simulink model "adaptive_sliding_mode_controller_computed_torque"  (R2020a)
settings: Solver=ode1  StartTime=0.0  StopTime=50  FixedStep=0.01  RelTol=1e-3
model workspace (MAT data in the model file):
  kd = 0
  kp = 0
libraries: simulink x19, sharedutil x14, aerolibutil x4
(part 1 of 2)
settings Model: Creator=Sebas  LastModifiedBy=Sebas
settings SolverCC: ZeroCrossAlgorithm=Adaptive
settings DebuggingCC: MaskedZcDiagnostic=none  IgnoredZcDiagnostic=none

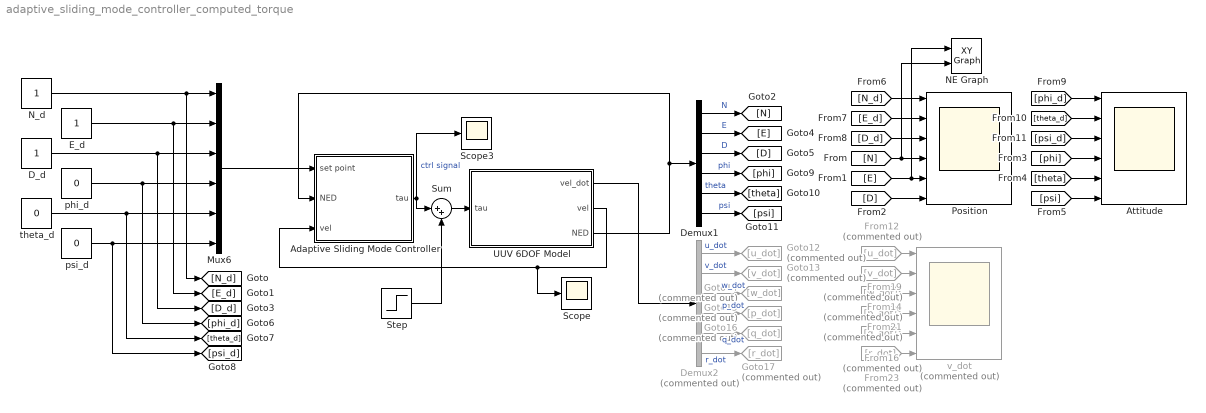
== system adaptive_sliding_mode_controller_computed_torque ==
  Adaptive Sliding Mode Controller : Subsystem
  Attitude : Scope  NumInputPorts=6
  D_d : Constant
  Demux1 : Demux  Outputs=6
  Demux2 : Demux  Commented=on  Outputs=6
  E_d : Constant
  From12 : From  Commented=on  GotoTag=u_dot
  From14 : From  Commented=on  GotoTag=w_dot
  From16 : From  Commented=on  GotoTag=q_dot
  From19 : From  Commented=on  GotoTag=v_dot
  From21 : From  Commented=on  GotoTag=p_dot
  From23 : From  Commented=on  GotoTag=r_dot
  Goto12 : Goto  Commented=on  GotoTag=u_dot
  Goto13 : Goto  Commented=on  GotoTag=v_dot
  Goto14 : Goto  Commented=on  GotoTag=w_dot
  Goto15 : Goto  Commented=on  GotoTag=p_dot
  Goto16 : Goto  Commented=on  GotoTag=q_dot
  Goto17 : Goto  Commented=on  GotoTag=r_dot
  Mux6 : Mux  Inputs=6
  NE Graph : simulink/Sinks/XY Graph  xmin=-1  xmax=5  ymin=-1  ymax=2  st=-1
  N_d : Constant
  Position : Scope  NumInputPorts=6
  Scope : Scope
  Scope3 : Scope
  Step : Step  Time=20  After=[30;30;30;5;5;5]  SampleTime=0
  Sum : Sum  Inputs=|++
  UUV 6DOF Model : Subsystem
  phi_d : Constant  Value=0
  psi_d : Constant  Value=0
  theta_d : Constant  Value=0
  v_dot : Scope  Commented=on  NumInputPorts=6
  wires:
  UUV 6DOF Model/3(NED) -> Adaptive Sliding Mode Controller/2(NED), Demux1/1
  Adaptive Sliding Mode Controller/1(tau) -> Sum/1, Scope3/1  "ctrl signal"
  [N_d] -> Position/1
  [E_d] -> Position/2
  [D_d] -> Position/3
  [N] -> Position/4, NE Graph/2
  [D] -> Position/6
  [E] -> Position/5, NE Graph/1
  Demux1/1 -> [N]  "N"
  Demux1/2 -> [E]  "E"
  Demux1/3 -> [D]  "D"
  [phi_d] -> Attitude/1
  [phi] -> Attitude/4
  [psi_d] -> Attitude/3
  [theta] -> Attitude/5
  [psi] -> Attitude/6
  [theta_d] -> Attitude/2
  Demux1/4 -> [phi]  "phi"
  Demux1/5 -> [theta]  "theta"
  Demux1/6 -> [psi]  "psi"
  UUV 6DOF Model/2(vel) -> Adaptive Sliding Mode Controller/3(vel), Scope/1
  UUV 6DOF Model/1(vel_dot) -> Demux2/1
  From12/1 -> v_dot/1
  From19/1 -> v_dot/2
  From14/1 -> v_dot/3
  From21/1 -> v_dot/4
  From16/1 -> v_dot/5
  From23/1 -> v_dot/6
  Demux2/1 -> Goto12/1  "u_dot"
  Demux2/5 -> Goto16/1  "q_dot"
  Demux2/3 -> Goto14/1  "w_dot"
  Demux2/6 -> Goto17/1  "r_dot"
  Demux2/4 -> Goto15/1  "p_dot"
  Demux2/2 -> Goto13/1  "v_dot"
  D_d/1 -> Mux6/3, [D_d]
  theta_d/1 -> [theta_d], Mux6/5
  Mux6/1 -> Adaptive Sliding Mode Controller/1(set point)
  phi_d/1 -> Mux6/4, [phi_d]
  E_d/1 -> [E_d], Mux6/2
  N_d/1 -> [N_d], Mux6/1
  psi_d/1 -> [psi_d], Mux6/6
  Sum/1 -> UUV 6DOF Model/1(tau)
  Step/1 -> Sum/2

== system adaptive_sliding_mode_controller_computed_torque/Adaptive Sliding Mode Controller ==
  set point : Inport
  NED : Inport  Port=2
  vel : Inport  Port=3
  ASMCs : Subsystem  Commented=on  mask(6 DOF Sliding Mode Controller){surge_k=10, sway_k=10, heave_k=2, roll_k=13, pitch_k=1, yaw_k=25, lambda=1, Kmin=0.001, k_alpha=0.002, miu=0.01}
      mask prompts: surge_k "Surge"; sway_k "Sway"; heave_k "Heave"; roll_k "Roll"; pitch_k "Pitch"; yaw_k "Yaw"
      mask help: Implementation of 6 Sliding Mode Controllers for each degree of freedom
      mask DialogControl ParameterGroupVar Prompt: K2 Gains
      mask DialogControl Container3 Prompt: Adaptation Law for K1
  ASMCs1 : Subsystem  Commented=on  mask(6 DOF Sliding Mode Controller){surge_k=3, sway_k=3, heave_k=1, roll_k=5, pitch_k=1, yaw_k=20, lambda=1, Kmin=0.005, k_alpha=0.0019, miu=0.01}
      mask prompts: surge_k "Surge"; sway_k "Sway"; heave_k "Heave"; roll_k "Roll"; pitch_k "Pitch"; yaw_k "Yaw"
      mask help: Implementation of 6 Sliding Mode Controllers for each degree of freedom
      mask DialogControl ParameterGroupVar Prompt: K2 Gains
      mask DialogControl Container3 Prompt: Adaptation Law for K1
  ASMCs2 : Subsystem  mask(6 DOF Sliding Mode Controller){surge_k=1, sway_k=1, heave_k=1, roll_k=5, pitch_k=1, yaw_k=20, lambda=1, Kmin=0.0001, k_alpha=0.1, miu=0.01}
      mask prompts: surge_k "Surge"; sway_k "Sway"; heave_k "Heave"; roll_k "Roll"; pitch_k "Pitch"; yaw_k "Yaw"
      mask help: Implementation of 6 Sliding Mode Controllers for each degree of freedom
      mask DialogControl ParameterGroupVar Prompt: K2 Gains
      mask DialogControl Container3 Prompt: Adaptation Law for K1
  NED to body : Subsystem
  Signal Specification : SignalSpecification  Dimensions=6
  Thrust allocation : Subsystem
  tau : Outport
  wires:
  NED to body/1(Out1) -> ASMCs2/1("position_d ")
  NED/1 -> NED to body/2(NED)
  Signal Specification/1 -> tau/1  "ideal"
  NED to body/2(Out2) -> ASMCs2/2(position)
  Thrust allocation/1(tau) -> Signal Specification/1
  ASMCs2/1(i_tau) -> Thrust allocation/1(ideal_tau)  "ideal_tau"
  vel/1 -> ASMCs2/3(vel)
  set point/1 -> NED to body/1(set point)

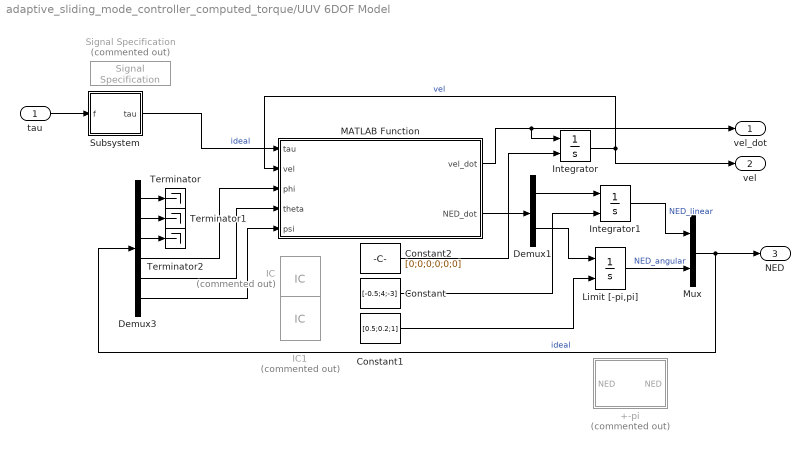
== system adaptive_sliding_mode_controller_computed_torque/UUV 6DOF Model ==
  tau : Inport
  +-pi : MATLAB Function  Commented=on  TreatAsAtomicUnit=on
  Constant : Constant  Value=[-0.5;4;-3]
  Constant1 : Constant  Value=[0.5;0.2;1]
  Constant2 : Constant  Value=[0;0;0;0;0;0]
  Demux1 : Demux  Outputs=2
  Demux3 : Demux  Outputs=6
  IC : InitialCondition  Commented=on  Value=[0;0;0;0;0;0]
  IC1 : InitialCondition  Commented=on  Value=[1;1;1;1;1;1]
  Integrator : Integrator  InitialConditionSource=external
  Integrator1 : Integrator  InitialConditionSource=external
  Limit [-pi,pi] : Integrator  InitialConditionSource=external  WrapState=on
  MATLAB Function : MATLAB Function  TreatAsAtomicUnit=on
  Mux : Mux  Inputs=2
  Signal Specification : SignalSpecification  Commented=on  Dimensions=6
  Subsystem : Subsystem
  Terminator : Terminator
  Terminator1 : Terminator
  Terminator2 : Terminator
  vel_dot : Outport
  vel : Outport  Port=2
  NED : Outport  Port=3
  wires:
  Constant/1 -> Integrator1/2
  Constant1/1 -> Limit [-pi,pi]/2
  Constant2/1 -> Integrator/2
  MATLAB Function/2(NED_dot) -> Demux1/1
  Demux1/1 -> Integrator1/1
  Demux1/2 -> Limit [-pi,pi]/1
  Limit [-pi,pi]/1 -> Mux/2  "NED_angular"
  tau/1 -> Subsystem/1(f)
  Subsystem/1(tau) -> MATLAB Function/1(tau)  "ideal"
  Demux3/3 -> Terminator2/1
  Demux3/1 -> Terminator/1
  Demux3/2 -> Terminator1/1
  Integrator1/1 -> Mux/1  "NED_linear"
  Demux3/6 -> MATLAB Function/5(psi)
  Demux3/5 -> MATLAB Function/4(theta)
  Demux3/4 -> MATLAB Function/3(phi)
  Integrator/1 -> MATLAB Function/2(vel), vel/1  "vel"
  MATLAB Function/1(vel_dot) -> Integrator/1, vel_dot/1
  Mux/1 -> NED/1, Demux3/1  "ideal"

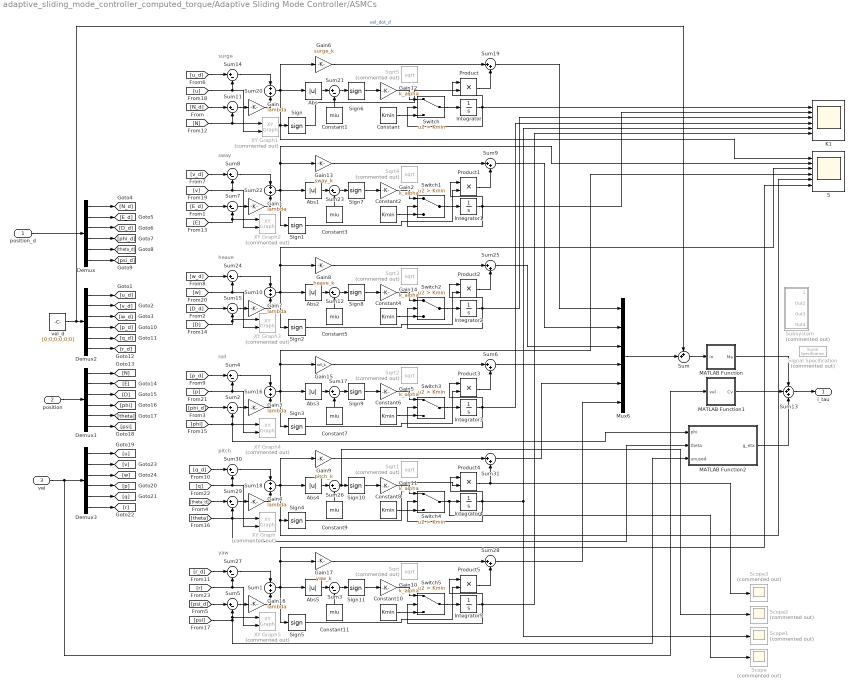
== system adaptive_sliding_mode_controller_computed_torque/Adaptive Sliding Mode Controller/ASMCs ==
  note: surge
  note: sway
  note: heave
  note: roll
  note: pitch
  note: yaw
  "position_d " : Inport
  position : Inport  Port=2
  vel : Inport  Port=3
  Abs{,1..5} (6 alike) : Abs
  Constant{,2,4,6,8,10} (6 alike) : Constant  Value=Kmin
  Constant{1,3,5,7,9,11} (6 alike) : Constant  Value=miu
  Demux{,1..3} (4 alike) : Demux  Outputs=6
  Gain{,1,3..4,7,16} (6 alike) : Gain  Gain=lambda
  Gain{2,5,10..12,14} (6 alike) : Gain  Gain=k_alpha
  Gain13 : Gain  Gain=sway_k
  Gain15 : Gain  Gain=roll_k
  Gain17 : Gain  Gain=yaw_k
  Gain6 : Gain  Gain=surge_k
  Gain8 : Gain  Gain=heave_k
  Gain9 : Gain  Gain=pitch_k
  Integrator{,1..5} (6 alike) : Integrator
  K1 : Scope  NumInputPorts=6
  MATLAB Function : MATLAB Function  TreatAsAtomicUnit=on
  MATLAB Function1 : MATLAB Function  TreatAsAtomicUnit=on
  MATLAB Function2 : MATLAB Function  TreatAsAtomicUnit=on
  Mux6 : Mux  Inputs=6
  Product{,1..5} (6 alike) : Product
  S : Scope  NumInputPorts=6
  Scope{,1..3} (4 alike) : Scope  Commented=on
  Sign{,1..11} (12 alike) : Signum  ZeroCross=off
  Signal Specification : SignalSpecification  Commented=on  Dimensions=6
  Sqrt{,1..5} (6 alike) : Sqrt  Commented=on  SaturateOnIntegerOverflow=on
  Subsystem : Subsystem  Commented=on
  Sum : Sum  Inputs=++|
  Sum{1,10,16,18,20,22} (6 alike) : Sum
  Sum{2..5,7..8,11..12,14..15,17,21,23..24,26..27,29..30} (18 alike) : Sum  Inputs=|+-
  Sum13 : Sum  Inputs=+++
  Sum{6,9,19,25,28,31} (6 alike) : Sum  Inputs=|++
  Switch{,1..5} (6 alike) : Switch  Criteria=u2 > Threshold  Threshold=Kmin
  XY Graph{,3..5} (4 alike) : simulink/Sinks/XY Graph  Commented=on  xmin=-1  xmax=1  ymin=-1  ymax=1  st=-1
  XY Graph1 : simulink/Sinks/XY Graph  Commented=on  xmin=-1  xmax=5  ymin=-1  ymax=1  st=-1
  XY Graph2 : simulink/Sinks/XY Graph  Commented=on  xmin=-1  xmax=5  ymin=-2  ymax=0.5  st=-1
  vel_d : Constant  Value=[0;0;0;0;0;0]
  i_tau : Outport
  wires:
  Sum25/1 -> Mux6/3
  Sum14/1 -> Sum20/1
  Sum11/1 -> Gain/1
  position/1 -> Demux1/1
  Demux1/1 -> [N]
  "position_d "/1 -> Demux/1
  Demux/1 -> [N_d]
  Demux1/2 -> [E]
  Demux/3 -> [D_d]
  Demux1/3 -> [D]
  Demux/4 -> [phi_d]
  Demux1/4 -> [phi]
  Demux/5 -> [theta_d]
  Demux1/5 -> [theta]
  Demux/6 -> [psi_d]
  Demux1/6 -> [psi]
  Sum/1 -> MATLAB Function/1(in)
  Sum13/1 -> i_tau/1
  vel/1 -> MATLAB Function1/1(vel), Demux3/1
  MATLAB Function2/1(g_eta) -> Sum13/3
  MATLAB Function1/1(Cv) -> Sum13/2
  Demux2/1 -> [u_d]
  Demux3/1 -> [u]
  Demux2/2 -> [v_d]
  Demux3/2 -> [v]
  Demux2/3 -> [w_d]
  Demux3/3 -> [w]
  Demux2/4 -> [p_d]
  Demux3/4 -> [p]
  Demux2/5 -> [q_d]
  Demux3/5 -> [q]
  Demux3/6 -> [r]
  Demux2/6 -> [r_d]
  [N_d] -> Sum11/1
  Demux/2 -> [E_d]
  [phi_d] -> Sum2/1
  [u_d] -> Sum14/1
  [p_d] -> Sum4/1
  [r_d] -> Sum27/1
  [N] -> XY Graph1/1, Sum11/2
  [theta] -> MATLAB Function2/2(theta), XY Graph/1, Sum29/2
  [u] -> Sum14/2, XY Graph1/2
  Gain/1 -> Sum20/2
  Sum20/1 -> S/1, Sign/1, Gain6/1, Abs/1
  Gain6/1 -> Sum19/1
  [v_d] -> Sum8/1
  [E_d] -> Sum7/1
  [w_d] -> Sum24/1
  [D_d] -> Sum15/1
  [q_d] -> Sum30/1
  [theta_d] -> Sum29/1
  vel_d/1 -> Sum/1, Demux2/1  "vel_dot_d"
  Mux6/1 -> Sum/2
  MATLAB Function/1(Ma) -> Sum13/1
  Sign/1 -> Product/2
  Switch/1 -> Integrator/1
  Integrator/1 -> Product/1, K1/1, Switch/2
  Constant/1 -> Switch/3
  Sign6/1 -> Gain12/1
  Abs/1 -> Sum21/1
  Constant1/1 -> Sum21/2
  Sum21/1 -> Sign6/1
  Gain12/1 -> Switch/1
  Product/1 -> Sum19/2
  Sum19/1 -> Mux6/1
  Product1/1 -> Sum9/2
  Gain2/1 -> Switch1/1
  Sum23/1 -> Sign7/1
  Constant3/1 -> Sum23/2
  Abs1/1 -> Sum23/1
  Sign7/1 -> Gain2/1
  Constant2/1 -> Switch1/3
  Integrator1/1 -> K1/2, Switch1/2, Product1/1
  Switch1/1 -> Integrator1/1
  Sign1/1 -> Product1/2
  Gain13/1 -> Sum9/1
  Sum22/1 -> S/2, Gain13/1, Abs1/1, Sign1/1
  Gain1/1 -> Sum22/2
  Sum7/1 -> Gain1/1
  Sum8/1 -> Sum22/1
  Sum9/1 -> Mux6/2
  Sum24/1 -> Sum10/1
  Sum15/1 -> Gain7/1
  Gain7/1 -> Sum10/2
  Sum10/1 -> S/3, Gain8/1, Sign2/1, Abs2/1
  Gain8/1 -> Sum25/1
  Sign2/1 -> Product2/2
  Switch2/1 -> Integrator2/1
  Integrator2/1 -> Product2/1, K1/3, Switch2/2
  Constant4/1 -> Switch2/3
  Sign8/1 -> Gain14/1
  Abs2/1 -> Sum12/1
  Constant5/1 -> Sum12/2
  Sum12/1 -> Sign8/1
  Gain14/1 -> Switch2/1
  Product2/1 -> Sum25/2
  [w] -> Sum24/2, XY Graph3/2
  [D] -> XY Graph3/1, Sum15/2
  [psi] -> XY Graph5/1, Sum5/2, MATLAB Function2/3(unused)
  [r] -> XY Graph5/2, Sum27/2
  Product5/1 -> Sum28/2
  Gain10/1 -> Switch5/1
  Sum3/1 -> Sign11/1
  Constant11/1 -> Sum3/2
  Abs5/1 -> Sum3/1
  Sign11/1 -> Gain10/1
  Constant10/1 -> Switch5/3
  Integrator5/1 -> Product5/1, K1/6, Switch5/2
  Switch5/1 -> Integrator5/1
  Sign5/1 -> Product5/2
  Gain17/1 -> Sum28/1
  Sum1/1 -> S/6, Gain17/1, Abs5/1, Sign5/1
  Gain16/1 -> Sum1/2
  Sum5/1 -> Gain16/1
  Sum27/1 -> Sum1/1
  Sum30/1 -> Sum18/1
  Sum29/1 -> Gain4/1
  Gain4/1 -> Sum18/2
  Sum18/1 -> S/5, Sign4/1, Abs4/1, Gain9/1
  Gain9/1 -> Sum31/1
  Sign4/1 -> Product4/2
  Switch4/1 -> Scope/1, Integrator4/1
  Integrator4/1 -> Product4/1, K1/5, Scope1/1, Switch4/2
  Constant8/1 -> Switch4/3
  Sign10/1 -> Gain11/1
  Abs4/1 -> Sum26/1
  Constant9/1 -> Sum26/2
  Sum26/1 -> Scope2/1, Sign10/1
  Gain11/1 -> Switch4/1
  Product4/1 -> Sum31/2, Scope3/1
  Product3/1 -> Sum6/2
  Gain5/1 -> Switch3/1
  Sum17/1 -> Sign9/1
  Constant7/1 -> Sum17/2
  Abs3/1 -> Sum17/1
  Sign9/1 -> Gain5/1
  Constant6/1 -> Switch3/3
  Integrator3/1 -> Product3/1, K1/4, Switch3/2
  Switch3/1 -> Integrator3/1
  Sign3/1 -> Product3/2
  Gain15/1 -> Sum6/1
  Sum16/1 -> S/4, Gain15/1, Abs3/1, Sign3/1
  Gain3/1 -> Sum16/2
  [p] -> Sum4/2, XY Graph4/2
  [phi] -> Sum2/2, XY Graph4/1, MATLAB Function2/1(phi)
  Sum2/1 -> Gain3/1
  Sum4/1 -> Sum16/1
  [psi_d] -> Sum5/1
  [q] -> Sum30/2, XY Graph/2
  Sum6/1 -> Mux6/4
  Sum31/1 -> Mux6/5
  Sum28/1 -> Mux6/6
  [v] -> XY Graph2/2, Sum8/2
  [E] -> XY Graph2/1, Sum7/2

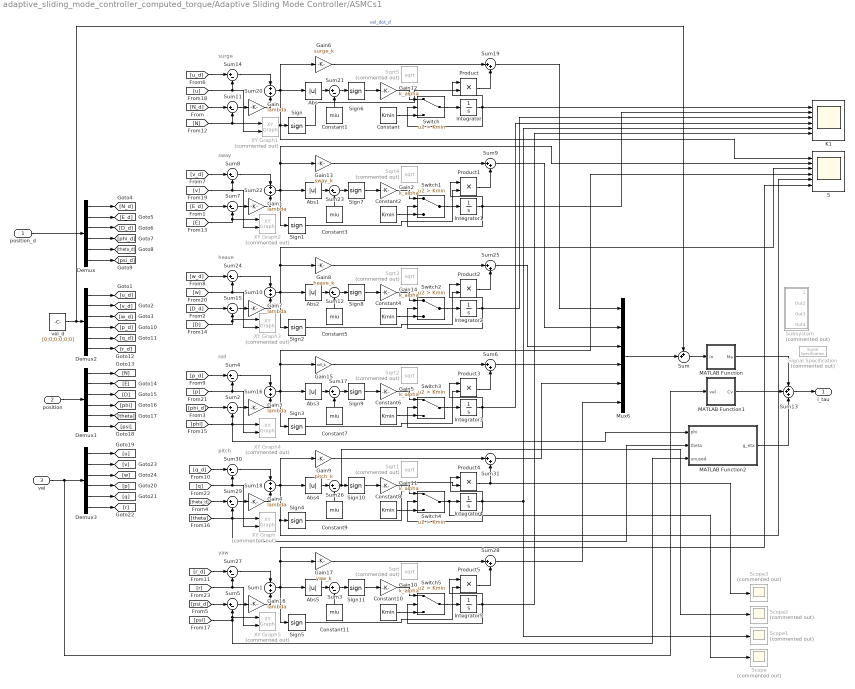
== system adaptive_sliding_mode_controller_computed_torque/Adaptive Sliding Mode Controller/ASMCs1 ==
  note: yaw
  note: pitch
  note: roll
  note: heave
  note: sway
  note: surge
  "position_d " : Inport
  position : Inport  Port=2
  vel : Inport  Port=3
  Abs{,1..5} (6 alike) : Abs
  Constant{,2,4,6,8,10} (6 alike) : Constant  Value=Kmin
  Constant{1,3,5,7,9,11} (6 alike) : Constant  Value=miu
  Demux{,1..3} (4 alike) : Demux  Outputs=6
  Gain{,1,3..4,7,16} (6 alike) : Gain  Gain=lambda
  Gain{2,5,10..12,14} (6 alike) : Gain  Gain=k_alpha
  Gain13 : Gain  Gain=sway_k
  Gain15 : Gain  Gain=roll_k
  Gain17 : Gain  Gain=yaw_k
  Gain6 : Gain  Gain=surge_k
  Gain8 : Gain  Gain=heave_k
  Gain9 : Gain  Gain=pitch_k
  Integrator{,1..5} (6 alike) : Integrator
  K1 : Scope  NumInputPorts=6
  MATLAB Function : MATLAB Function  TreatAsAtomicUnit=on
  MATLAB Function1 : MATLAB Function  TreatAsAtomicUnit=on
  MATLAB Function2 : MATLAB Function  TreatAsAtomicUnit=on
  Mux6 : Mux  Inputs=6
  Product{,1..5} (6 alike) : Product
  S : Scope  NumInputPorts=6
  Scope{,1..3} (4 alike) : Scope  Commented=on
  Sign{,1..11} (12 alike) : Signum  ZeroCross=off
  Signal Specification : SignalSpecification  Commented=on  Dimensions=6
  Sqrt{,1..5} (6 alike) : Sqrt  Commented=on  SaturateOnIntegerOverflow=on
  Subsystem : Subsystem  Commented=on
  Sum : Sum  Inputs=++|
  Sum{1,10,16,18,20,22} (6 alike) : Sum
  Sum{2..5,7..8,11..12,14..15,17,21,23..24,26..27,29..30} (18 alike) : Sum  Inputs=|+-
  Sum13 : Sum  Inputs=+++
  Sum{6,9,19,25,28,31} (6 alike) : Sum  Inputs=|++
  Switch{,1..5} (6 alike) : Switch  Criteria=u2 > Threshold  Threshold=Kmin
  XY Graph{,3..5} (4 alike) : simulink/Sinks/XY Graph  Commented=on  xmin=-1  xmax=1  ymin=-1  ymax=1  st=-1
  XY Graph1 : simulink/Sinks/XY Graph  Commented=on  xmin=-1  xmax=5  ymin=-1  ymax=1  st=-1
  XY Graph2 : simulink/Sinks/XY Graph  Commented=on  xmin=-1  xmax=5  ymin=-2  ymax=0.5  st=-1
  vel_d : Constant  Value=[0;0;0;0;0;0]
  i_tau : Outport
  wires:
  [E] -> Sum7/2, XY Graph2/1
  [v] -> Sum8/2, XY Graph2/2
  Sum28/1 -> Mux6/6
  Sum31/1 -> Mux6/5
  Sum6/1 -> Mux6/4
  [q] -> XY Graph/2, Sum30/2
  [psi_d] -> Sum5/1
  Sum4/1 -> Sum16/1
  Sum2/1 -> Gain3/1
  [phi] -> MATLAB Function2/1(phi), XY Graph4/1, Sum2/2
  [p] -> XY Graph4/2, Sum4/2
  Gain3/1 -> Sum16/2
  Sum16/1 -> Sign3/1, Abs3/1, Gain15/1, S/4
  Gain15/1 -> Sum6/1
  Sign3/1 -> Product3/2
  Switch3/1 -> Integrator3/1
  Integrator3/1 -> Switch3/2, K1/4, Product3/1
  Constant6/1 -> Switch3/3
  Sign9/1 -> Gain5/1
  Abs3/1 -> Sum17/1
  Constant7/1 -> Sum17/2
  Sum17/1 -> Sign9/1
  Gain5/1 -> Switch3/1
  Product3/1 -> Sum6/2
  Product4/1 -> Scope3/1, Sum31/2
  Gain11/1 -> Switch4/1
  Sum26/1 -> Sign10/1, Scope2/1
  Constant9/1 -> Sum26/2
  Abs4/1 -> Sum26/1
  Sign10/1 -> Gain11/1
  Constant8/1 -> Switch4/3
  Integrator4/1 -> Switch4/2, Scope1/1, K1/5, Product4/1
  Switch4/1 -> Integrator4/1, Scope/1
  Sign4/1 -> Product4/2
  Gain9/1 -> Sum31/1
  Sum18/1 -> Gain9/1, Abs4/1, Sign4/1, S/5
  Gain4/1 -> Sum18/2
  Sum29/1 -> Gain4/1
  Sum30/1 -> Sum18/1
  Sum27/1 -> Sum1/1
  Sum5/1 -> Gain16/1
  Gain16/1 -> Sum1/2
  Sum1/1 -> Sign5/1, Abs5/1, Gain17/1, S/6
  Gain17/1 -> Sum28/1
  Sign5/1 -> Product5/2
  Switch5/1 -> Integrator5/1
  Integrator5/1 -> Switch5/2, K1/6, Product5/1
  Constant10/1 -> Switch5/3
  Sign11/1 -> Gain10/1
  Abs5/1 -> Sum3/1
  Constant11/1 -> Sum3/2
  Sum3/1 -> Sign11/1
  Gain10/1 -> Switch5/1
  Product5/1 -> Sum28/2
  [r] -> Sum27/2, XY Graph5/2
  [psi] -> MATLAB Function2/3(unused), Sum5/2, XY Graph5/1
  [D] -> Sum15/2, XY Graph3/1
  [w] -> XY Graph3/2, Sum24/2
  Product2/1 -> Sum25/2
  Gain14/1 -> Switch2/1
  Sum12/1 -> Sign8/1
  Constant5/1 -> Sum12/2
  Abs2/1 -> Sum12/1
  Sign8/1 -> Gain14/1
  Constant4/1 -> Switch2/3
  Integrator2/1 -> Switch2/2, K1/3, Product2/1
  Switch2/1 -> Integrator2/1
  Sign2/1 -> Product2/2
  Gain8/1 -> Sum25/1
  Sum10/1 -> Abs2/1, Sign2/1, Gain8/1, S/3
  Gain7/1 -> Sum10/2
  Sum15/1 -> Gain7/1
  Sum24/1 -> Sum10/1
  Sum9/1 -> Mux6/2
  Sum8/1 -> Sum22/1
  Sum7/1 -> Gain1/1
  Gain1/1 -> Sum22/2
  Sum22/1 -> Sign1/1, Abs1/1, Gain13/1, S/2
  Gain13/1 -> Sum9/1
  Sign1/1 -> Product1/2
  Switch1/1 -> Integrator1/1
  Integrator1/1 -> Product1/1, Switch1/2, K1/2
  Constant2/1 -> Switch1/3
  Sign7/1 -> Gain2/1
  Abs1/1 -> Sum23/1
  Constant3/1 -> Sum23/2
  Sum23/1 -> Sign7/1
  Gain2/1 -> Switch1/1
  Product1/1 -> Sum9/2
  Sum19/1 -> Mux6/1
  Product/1 -> Sum19/2
  Gain12/1 -> Switch/1
  Sum21/1 -> Sign6/1
  Constant1/1 -> Sum21/2
  Abs/1 -> Sum21/1
  Sign6/1 -> Gain12/1
  Constant/1 -> Switch/3
  Integrator/1 -> Switch/2, K1/1, Product/1
  Switch/1 -> Integrator/1
  Sign/1 -> Product/2
  MATLAB Function/1(Ma) -> Sum13/1
  Mux6/1 -> Sum/2
  vel_d/1 -> Demux2/1, Sum/1  "vel_dot_d"
  [theta_d] -> Sum29/1
  [q_d] -> Sum30/1
  [D_d] -> Sum15/1
  [w_d] -> Sum24/1
  [E_d] -> Sum7/1
  [v_d] -> Sum8/1
  Gain6/1 -> Sum19/1
  Sum20/1 -> Abs/1, Gain6/1, Sign/1, S/1
  Gain/1 -> Sum20/2
  [u] -> XY Graph1/2, Sum14/2
  [theta] -> Sum29/2, XY Graph/1, MATLAB Function2/2(theta)
  [N] -> Sum11/2, XY Graph1/1
  [r_d] -> Sum27/1
  [p_d] -> Sum4/1
  [u_d] -> Sum14/1
  [phi_d] -> Sum2/1
  Demux/2 -> [E_d]
  [N_d] -> Sum11/1
  Demux2/6 -> [r_d]
  Demux3/6 -> [r]
  Demux3/5 -> [q]
  Demux2/5 -> [q_d]
  Demux3/4 -> [p]
  Demux2/4 -> [p_d]
  Demux3/3 -> [w]
  Demux2/3 -> [w_d]
  Demux3/2 -> [v]
  Demux2/2 -> [v_d]
  Demux3/1 -> [u]
  Demux2/1 -> [u_d]
  MATLAB Function1/1(Cv) -> Sum13/2
  MATLAB Function2/1(g_eta) -> Sum13/3
  vel/1 -> Demux3/1, MATLAB Function1/1(vel)
  Sum13/1 -> i_tau/1
  Sum/1 -> MATLAB Function/1(in)
  Demux1/6 -> [psi]
  Demux/6 -> [psi_d]
  Demux1/5 -> [theta]
  Demux/5 -> [theta_d]
  Demux1/4 -> [phi]
  Demux/4 -> [phi_d]
  Demux1/3 -> [D]
  Demux/3 -> [D_d]
  Demux1/2 -> [E]
  Demux/1 -> [N_d]
  "position_d "/1 -> Demux/1
  Demux1/1 -> [N]
  position/1 -> Demux1/1
  Sum11/1 -> Gain/1
  Sum14/1 -> Sum20/1
  Sum25/1 -> Mux6/3

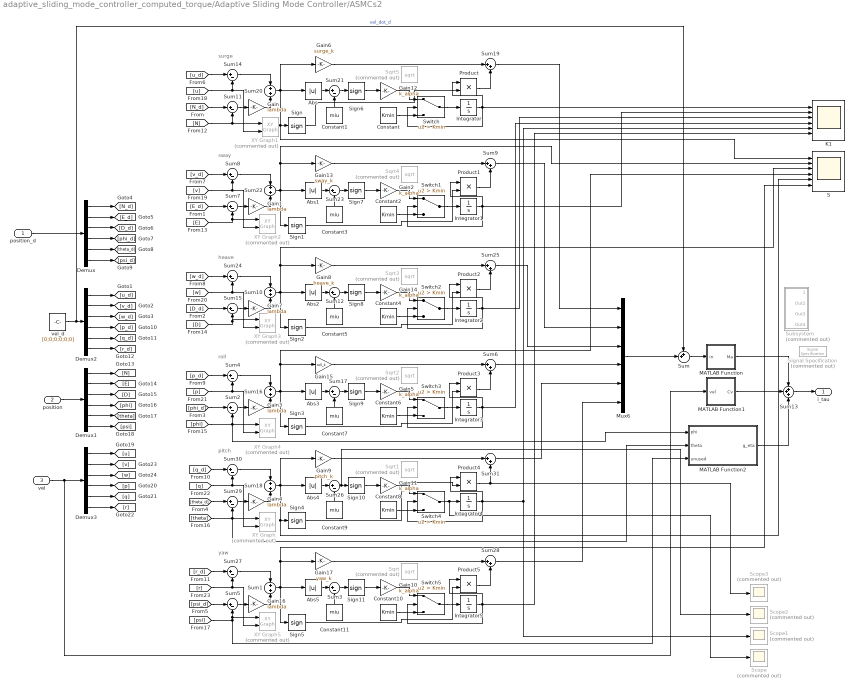
== system adaptive_sliding_mode_controller_computed_torque/Adaptive Sliding Mode Controller/ASMCs2 ==
  note: surge
  note: sway
  note: heave
  note: roll
  note: pitch
  note: yaw
  "position_d " : Inport
  position : Inport  Port=2
  vel : Inport  Port=3
  Abs{,1..5} (6 alike) : Abs
  Constant{,2,4,6,8,10} (6 alike) : Constant  Value=Kmin
  Constant{1,3,5,7,9,11} (6 alike) : Constant  Value=miu
  Demux{,1..3} (4 alike) : Demux  Outputs=6
  Gain{,1,3..4,7,16} (6 alike) : Gain  Gain=lambda
  Gain{2,5,10..12,14} (6 alike) : Gain  Gain=k_alpha
  Gain13 : Gain  Gain=sway_k
  Gain15 : Gain  Gain=roll_k
  Gain17 : Gain  Gain=yaw_k
  Gain6 : Gain  Gain=surge_k
  Gain8 : Gain  Gain=heave_k
  Gain9 : Gain  Gain=pitch_k
  Integrator{,1..5} (6 alike) : Integrator
  K1 : Scope  NumInputPorts=6
  MATLAB Function : MATLAB Function  TreatAsAtomicUnit=on
  MATLAB Function1 : MATLAB Function  TreatAsAtomicUnit=on
  MATLAB Function2 : MATLAB Function  TreatAsAtomicUnit=on
  Mux6 : Mux  Inputs=6
  Product{,1..5} (6 alike) : Product
  S : Scope  NumInputPorts=6
  Scope{,1..3} (4 alike) : Scope  Commented=on
  Sign{,1..11} (12 alike) : Signum  ZeroCross=off
  Signal Specification : SignalSpecification  Commented=on  Dimensions=6
  Sqrt{,1..5} (6 alike) : Sqrt  Commented=on  SaturateOnIntegerOverflow=on
  Subsystem : Subsystem  Commented=on
  Sum : Sum  Inputs=++|
  Sum{1,10,16,18,20,22} (6 alike) : Sum
  Sum{2..5,7..8,11..12,14..15,17,21,23..24,26..27,29..30} (18 alike) : Sum  Inputs=|+-
  Sum13 : Sum  Inputs=+++
  Sum{6,9,19,25,28,31} (6 alike) : Sum  Inputs=|++
  Switch{,1..5} (6 alike) : Switch  Criteria=u2 > Threshold  Threshold=Kmin
  XY Graph{,3..5} (4 alike) : simulink/Sinks/XY Graph  Commented=on  xmin=-1  xmax=1  ymin=-1  ymax=1  st=-1
  XY Graph1 : simulink/Sinks/XY Graph  Commented=on  xmin=-1  xmax=5  ymin=-1  ymax=1  st=-1
  XY Graph2 : simulink/Sinks/XY Graph  Commented=on  xmin=-1  xmax=5  ymin=-2  ymax=0.5  st=-1
  vel_d : Constant  Value=[0;0;0;0;0;0]
  i_tau : Outport
  wires:
  Sum25/1 -> Mux6/3
  Sum14/1 -> Sum20/1
  Sum11/1 -> Gain/1
  position/1 -> Demux1/1
  Demux1/1 -> [N]
  "position_d "/1 -> Demux/1
  Demux/1 -> [N_d]
  Demux1/2 -> [E]
  Demux/3 -> [D_d]
  Demux1/3 -> [D]
  Demux/4 -> [phi_d]
  Demux1/4 -> [phi]
  Demux/5 -> [theta_d]
  Demux1/5 -> [theta]
  Demux/6 -> [psi_d]
  Demux1/6 -> [psi]
  Sum/1 -> MATLAB Function/1(in)
  Sum13/1 -> i_tau/1
  vel/1 -> MATLAB Function1/1(vel), Demux3/1
  MATLAB Function2/1(g_eta) -> Sum13/3
  MATLAB Function1/1(Cv) -> Sum13/2
  Demux2/1 -> [u_d]
  Demux3/1 -> [u]
  Demux2/2 -> [v_d]
  Demux3/2 -> [v]
  Demux2/3 -> [w_d]
  Demux3/3 -> [w]
  Demux2/4 -> [p_d]
  Demux3/4 -> [p]
  Demux2/5 -> [q_d]
  Demux3/5 -> [q]
  Demux3/6 -> [r]
  Demux2/6 -> [r_d]
  [N_d] -> Sum11/1
  Demux/2 -> [E_d]
  [phi_d] -> Sum2/1
  [u_d] -> Sum14/1
  [p_d] -> Sum4/1
  [r_d] -> Sum27/1
  [N] -> XY Graph1/1, Sum11/2
  [theta] -> MATLAB Function2/2(theta), XY Graph/1, Sum29/2
  [u] -> Sum14/2, XY Graph1/2
  Gain/1 -> Sum20/2
  Sum20/1 -> S/1, Sign/1, Gain6/1, Abs/1
  Gain6/1 -> Sum19/1
  [v_d] -> Sum8/1
  [E_d] -> Sum7/1
  [w_d] -> Sum24/1
  [D_d] -> Sum15/1
  [q_d] -> Sum30/1
  [theta_d] -> Sum29/1
  vel_d/1 -> Sum/1, Demux2/1  "vel_dot_d"
  Mux6/1 -> Sum/2
  MATLAB Function/1(Ma) -> Sum13/1
  Sign/1 -> Product/2
  Switch/1 -> Integrator/1
  Integrator/1 -> Product/1, K1/1, Switch/2
  Constant/1 -> Switch/3
  Sign6/1 -> Gain12/1
  Abs/1 -> Sum21/1
  Constant1/1 -> Sum21/2
  Sum21/1 -> Sign6/1
  Gain12/1 -> Switch/1
  Product/1 -> Sum19/2
  Sum19/1 -> Mux6/1
  Product1/1 -> Sum9/2
  Gain2/1 -> Switch1/1
  Sum23/1 -> Sign7/1
  Constant3/1 -> Sum23/2
  Abs1/1 -> Sum23/1
  Sign7/1 -> Gain2/1
  Constant2/1 -> Switch1/3
  Integrator1/1 -> K1/2, Switch1/2, Product1/1
  Switch1/1 -> Integrator1/1
  Sign1/1 -> Product1/2
  Gain13/1 -> Sum9/1
  Sum22/1 -> S/2, Gain13/1, Abs1/1, Sign1/1
  Gain1/1 -> Sum22/2
  Sum7/1 -> Gain1/1
  Sum8/1 -> Sum22/1
  Sum9/1 -> Mux6/2
  Sum24/1 -> Sum10/1
  Sum15/1 -> Gain7/1
  Gain7/1 -> Sum10/2
  Sum10/1 -> S/3, Gain8/1, Sign2/1, Abs2/1
  Gain8/1 -> Sum25/1
  Sign2/1 -> Product2/2
  Switch2/1 -> Integrator2/1
  Integrator2/1 -> Product2/1, K1/3, Switch2/2
  Constant4/1 -> Switch2/3
  Sign8/1 -> Gain14/1
  Abs2/1 -> Sum12/1
  Constant5/1 -> Sum12/2
  Sum12/1 -> Sign8/1
  Gain14/1 -> Switch2/1
  Product2/1 -> Sum25/2
  [w] -> Sum24/2, XY Graph3/2
  [D] -> XY Graph3/1, Sum15/2
  [psi] -> XY Graph5/1, Sum5/2, MATLAB Function2/3(unused)
  [r] -> XY Graph5/2, Sum27/2
  Product5/1 -> Sum28/2
  Gain10/1 -> Switch5/1
  Sum3/1 -> Sign11/1
  Constant11/1 -> Sum3/2
  Abs5/1 -> Sum3/1
  Sign11/1 -> Gain10/1
  Constant10/1 -> Switch5/3
  Integrator5/1 -> Product5/1, K1/6, Switch5/2
  Switch5/1 -> Integrator5/1
  Sign5/1 -> Product5/2
  Gain17/1 -> Sum28/1
  Sum1/1 -> S/6, Gain17/1, Abs5/1, Sign5/1
  Gain16/1 -> Sum1/2
  Sum5/1 -> Gain16/1
  Sum27/1 -> Sum1/1
  Sum30/1 -> Sum18/1
  Sum29/1 -> Gain4/1
  Gain4/1 -> Sum18/2
  Sum18/1 -> S/5, Sign4/1, Abs4/1, Gain9/1
  Gain9/1 -> Sum31/1
  Sign4/1 -> Product4/2
  Switch4/1 -> Scope/1, Integrator4/1
  Integrator4/1 -> Product4/1, K1/5, Scope1/1, Switch4/2
  Constant8/1 -> Switch4/3
  Sign10/1 -> Gain11/1
  Abs4/1 -> Sum26/1
  Constant9/1 -> Sum26/2
  Sum26/1 -> Scope2/1, Sign10/1
  Gain11/1 -> Switch4/1
  Product4/1 -> Sum31/2, Scope3/1
  Product3/1 -> Sum6/2
  Gain5/1 -> Switch3/1
  Sum17/1 -> Sign9/1
  Constant7/1 -> Sum17/2
  Abs3/1 -> Sum17/1
  Sign9/1 -> Gain5/1
  Constant6/1 -> Switch3/3
  Integrator3/1 -> Product3/1, K1/4, Switch3/2
  Switch3/1 -> Integrator3/1
  Sign3/1 -> Product3/2
  Gain15/1 -> Sum6/1
  Sum16/1 -> S/4, Gain15/1, Abs3/1, Sign3/1
  Gain3/1 -> Sum16/2
  [p] -> Sum4/2, XY Graph4/2
  [phi] -> Sum2/2, XY Graph4/1, MATLAB Function2/1(phi)
  Sum2/1 -> Gain3/1
  Sum4/1 -> Sum16/1
  [psi_d] -> Sum5/1
  [q] -> Sum30/2, XY Graph/2
  Sum6/1 -> Mux6/4
  Sum31/1 -> Mux6/5
  Sum28/1 -> Mux6/6
  [v] -> XY Graph2/2, Sum8/2
  [E] -> XY Graph2/1, Sum7/2

== system adaptive_sliding_mode_controller_computed_torque/Adaptive Sliding Mode Controller/NED to body ==
  set point : Inport
  NED : Inport  Port=2
  Demux : Demux  Outputs=2
  Demux1 : Demux  Outputs=2
  Mux1 : Mux  Inputs=2
  Mux2 : Mux  Inputs=2
  Mux3 : Mux  Inputs=2
  Subsystem1 : Subsystem
  Subsystem2 : Subsystem
  Terminator5 : Terminator
  Out1 : Outport
  Out2 : Outport  Port=2
  wires:
  Demux/1 -> Mux2/1
  NED/1 -> Demux1/1, Subsystem1/1(NED)
  set point/1 -> Demux/1
  Demux/2 -> Mux1/2
  Subsystem2/1(pos_body) -> Mux1/1
  Demux1/1 -> Terminator5/1
  Subsystem1/1(pos_body) -> Mux3/1
  Demux1/2 -> Mux2/2, Mux3/2
  Mux2/1 -> Subsystem2/1(NED)
  Mux3/1 -> Out2/1
  Mux1/1 -> Out1/1

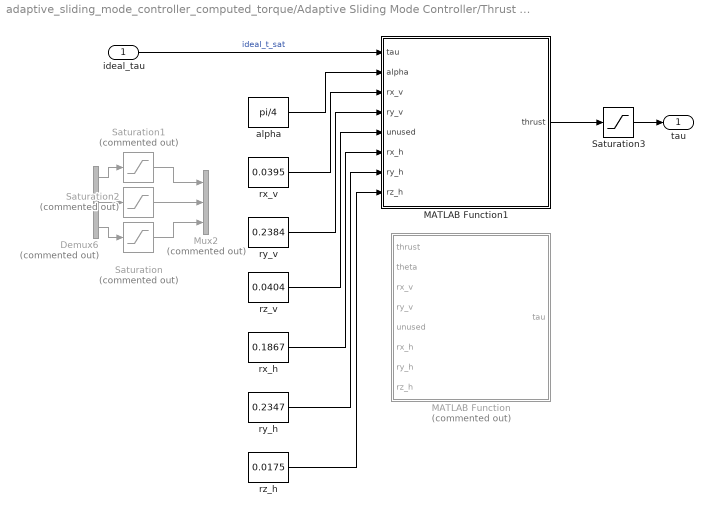
== system adaptive_sliding_mode_controller_computed_torque/Adaptive Sliding Mode Controller/Thrust allocation ==
  ideal_tau : Inport
  Demux6 : Demux  Commented=on  Outputs=3
  MATLAB Function : MATLAB Function  Commented=on  TreatAsAtomicUnit=on
  MATLAB Function1 : MATLAB Function  TreatAsAtomicUnit=on
  Mux2 : Mux  Commented=on  Inputs=3
  Saturation : Saturate  Commented=on  UpperLimit=70  LowerLimit=-70
  Saturation1 : Saturate  Commented=on  UpperLimit=100  LowerLimit=-100
  Saturation2 : Saturate  Commented=on  UpperLimit=100  LowerLimit=-100
  Saturation3 : Saturate  UpperLimit=35  LowerLimit=-35
  alpha : Constant  Value=pi/4
  rx_h : Constant  Value=0.1867
  rx_v : Constant  Value=0.0395
  ry_h : Constant  Value=0.2347
  ry_v : Constant  Value=0.2384
  rz_h : Constant  Value=0.0175
  rz_v : Constant  Value=0.0404
  tau : Outport
  wires:
  ideal_tau/1 -> MATLAB Function1/1(tau)  "ideal_t_sat"
  MATLAB Function1/1(thrust) -> Saturation3/1
  Saturation3/1 -> tau/1
  rx_v/1 -> MATLAB Function1/3(rx_v)
  alpha/1 -> MATLAB Function1/2(alpha)
  rx_h/1 -> MATLAB Function1/6(rx_h)
  ry_h/1 -> MATLAB Function1/7(ry_h)
  rz_h/1 -> MATLAB Function1/8(rz_h)
  ry_v/1 -> MATLAB Function1/4(ry_v)
  rz_v/1 -> MATLAB Function1/5(unused)
  Demux6/2 -> Saturation2/1
  Demux6/3 -> Saturation/1
  Saturation1/1 -> Mux2/1
  Saturation/1 -> Mux2/3
  Demux6/1 -> Saturation1/1
  Saturation2/1 -> Mux2/2

== system adaptive_sliding_mode_controller_computed_torque/UUV 6DOF Model/Subsystem ==
  f : Inport
  MATLAB Function1 : MATLAB Function  TreatAsAtomicUnit=on
  rx_h : Constant  Value=0.1867
  rx_v : Constant  Value=0.0395
  ry_h : Constant  Value=0.2347
  ry_v : Constant  Value=0.2384
  rz_h : Constant  Value=0.0175
  rz_v : Constant  Value=0.0404
  theta : Constant  Value=pi/4
  tau : Outport
  wires:
  rz_v/1 -> MATLAB Function1/5(unused)
  ry_h/1 -> MATLAB Function1/7(ry_h)
  f/1 -> MATLAB Function1/1(f)
  MATLAB Function1/1(tau) -> tau/1
  rx_h/1 -> MATLAB Function1/6(rx_h)
  theta/1 -> MATLAB Function1/2(theta)
  rx_v/1 -> MATLAB Function1/3(rx_v)
  rz_h/1 -> MATLAB Function1/8(rz_h)
  ry_v/1 -> MATLAB Function1/4(ry_v)

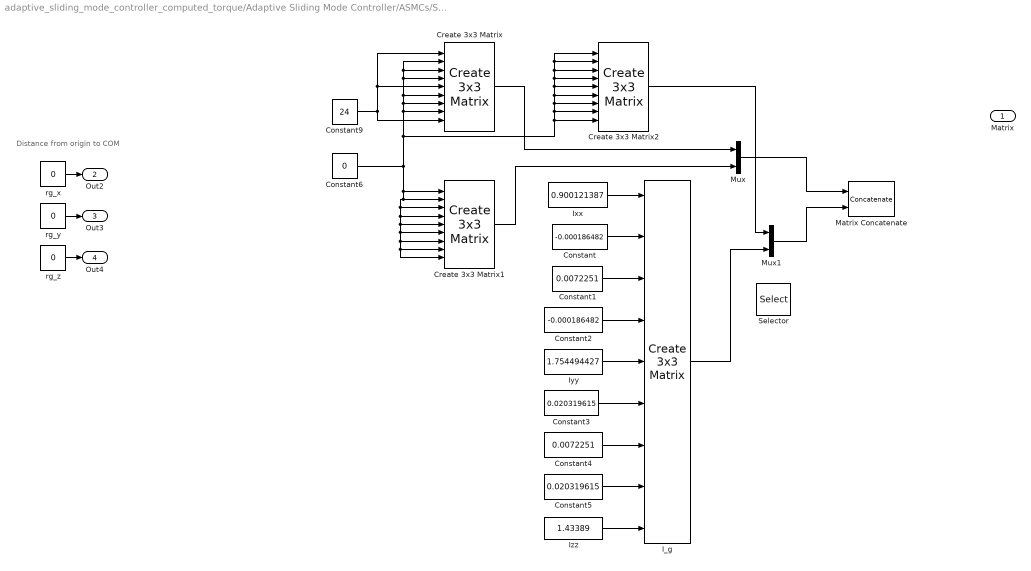
== system adaptive_sliding_mode_controller_computed_torque/Adaptive Sliding Mode Controller/ASMCs/Subsystem ==
  note: Distance from origin to COM
  Constant : Constant  Value=-0.000186482
  Constant1 : Constant  Value=0.0072251
  Constant2 : Constant  Value=-0.000186482
  Constant3 : Constant  Value=0.020319615
  Constant4 : Constant  Value=0.0072251
  Constant5 : Constant  Value=0.020319615
  Constant6 : Constant  Value=0
  Constant9 : Constant  Value=24
  Create 3x3 Matrix : sharedutil/Create 3x3 Matrix  aMode=aMode
      settings: SourceProductBaseCode=AE,PW,MT,VE,VP
  Create 3x3 Matrix1 : sharedutil/Create 3x3 Matrix  aMode=aMode
      settings: SourceProductBaseCode=AE,PW,MT,VE,VP
  Create 3x3 Matrix2 : sharedutil/Create 3x3 Matrix  aMode=aMode
      settings: SourceProductBaseCode=AE,PW,MT,VE,VP
  I_g : sharedutil/Create 3x3 Matrix  aMode=aMode
      settings: SourceProductBaseCode=AE,PW,MT,VE,VP
  Ixx : Constant  Value=0.900121387
  Iyy : Constant  Value=1.754494427
  Izz : Constant  Value=1.43389
  Matrix Concatenate : Concatenate  Mode=Multidimensional array  ConcatenateDimension=2
  Mux : Mux  Inputs=2
  Mux1 : Mux  Inputs=2
  Selector : Selector  InputPortWidth=3  IndexOptions=Index vector (dialog)  Indices=[1 3]  OutputSizes=1
  rg_x : Constant  Value=0
  rg_y : Constant  Value=0
  rg_z : Constant  Value=0
  Matrix : Outport
  Out2 : Outport  Port=2
  Out3 : Outport  Port=3
  Out4 : Outport  Port=4
  wires:
  Constant1/1 -> I_g/3
  Constant4/1 -> I_g/7
  Ixx/1 -> I_g/1
  rg_z/1 -> Out4/1
  Constant/1 -> I_g/2
  Constant5/1 -> I_g/8
  Constant2/1 -> I_g/4
  Constant3/1 -> I_g/6
  Iyy/1 -> I_g/5
  Izz/1 -> I_g/9
  rg_x/1 -> Out2/1
  rg_y/1 -> Out3/1
  Constant9/1 -> Create 3x3 Matrix/9, Create 3x3 Matrix/1, Create 3x3 Matrix/5
  Create 3x3 Matrix/1 -> Mux/1
  Create 3x3 Matrix1/1 -> Mux/2
  Constant6/1 -> Create 3x3 Matrix2/1, Create 3x3 Matrix2/2, Create 3x3 Matrix2/3, Create 3x3 Matrix2/4, Create 3x3 Matrix2/5, Create 3x3 Matrix2/6, Create 3x3 Matrix2/7, Create 3x3 Matrix2/8, Create 3x3 Matrix2/9, Create 3x3 Matrix/2, Create 3x3 Matrix/3, Create 3x3 Matrix/4, Create 3x3 Matrix/6, Create 3x3 Matrix/7, Create 3x3 Matrix/8, Create 3x3 Matrix1/2, Create 3x3 Matrix1/3, Create 3x3 Matrix1/8, Create 3x3 Matrix1/9, Create 3x3 Matrix1/7, Create 3x3 Matrix1/6, Create 3x3 Matrix1/5, Create 3x3 Matrix1/4, Create 3x3 Matrix1/1
  Create 3x3 Matrix2/1 -> Mux1/1
  I_g/1 -> Mux1/2
  Mux/1 -> Matrix Concatenate/1
  Mux1/1 -> Matrix Concatenate/2

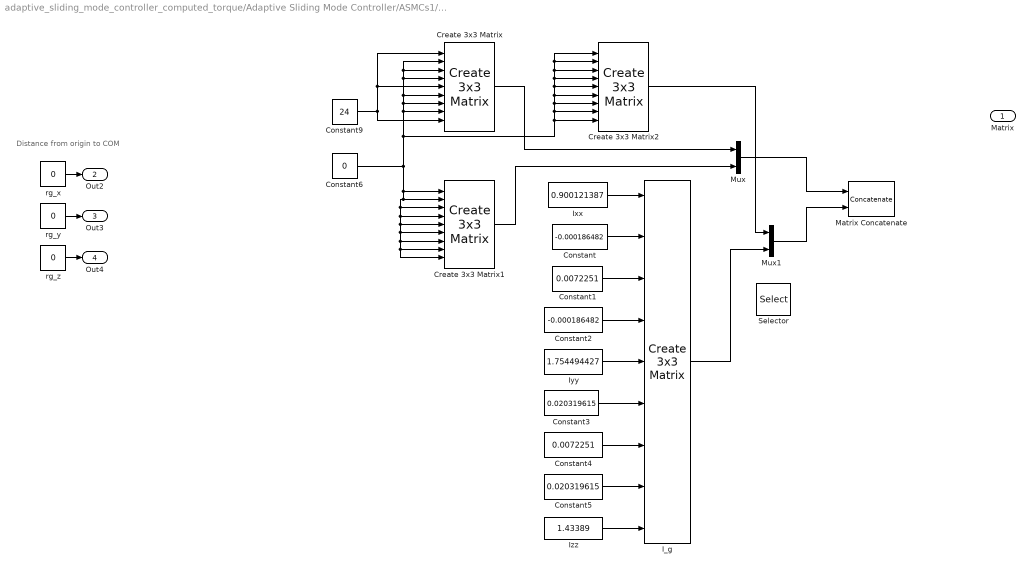
== system adaptive_sliding_mode_controller_computed_torque/Adaptive Sliding Mode Controller/ASMCs1/Subsystem ==
  note: Distance from origin to COM
  Constant : Constant  Value=-0.000186482
  Constant1 : Constant  Value=0.0072251
  Constant2 : Constant  Value=-0.000186482
  Constant3 : Constant  Value=0.020319615
  Constant4 : Constant  Value=0.0072251
  Constant5 : Constant  Value=0.020319615
  Constant6 : Constant  Value=0
  Constant9 : Constant  Value=24
  Create 3x3 Matrix : sharedutil/Create 3x3 Matrix  aMode=aMode
      settings: SourceProductBaseCode=AE,PW,MT,VE,VP
  Create 3x3 Matrix1 : sharedutil/Create 3x3 Matrix  aMode=aMode
      settings: SourceProductBaseCode=AE,PW,MT,VE,VP
  Create 3x3 Matrix2 : sharedutil/Create 3x3 Matrix  aMode=aMode
      settings: SourceProductBaseCode=AE,PW,MT,VE,VP
  I_g : sharedutil/Create 3x3 Matrix  aMode=aMode
      settings: SourceProductBaseCode=AE,PW,MT,VE,VP
  Ixx : Constant  Value=0.900121387
  Iyy : Constant  Value=1.754494427
  Izz : Constant  Value=1.43389
  Matrix Concatenate : Concatenate  Mode=Multidimensional array  ConcatenateDimension=2
  Mux : Mux  Inputs=2
  Mux1 : Mux  Inputs=2
  Selector : Selector  InputPortWidth=3  IndexOptions=Index vector (dialog)  Indices=[1 3]  OutputSizes=1
  rg_x : Constant  Value=0
  rg_y : Constant  Value=0
  rg_z : Constant  Value=0
  Matrix : Outport
  Out2 : Outport  Port=2
  Out3 : Outport  Port=3
  Out4 : Outport  Port=4
  wires:
  Mux1/1 -> Matrix Concatenate/2
  Mux/1 -> Matrix Concatenate/1
  I_g/1 -> Mux1/2
  Create 3x3 Matrix2/1 -> Mux1/1
  Constant6/1 -> Create 3x3 Matrix1/1, Create 3x3 Matrix1/4, Create 3x3 Matrix1/5, Create 3x3 Matrix1/6, Create 3x3 Matrix1/7, Create 3x3 Matrix1/9, Create 3x3 Matrix1/8, Create 3x3 Matrix1/3, Create 3x3 Matrix1/2, Create 3x3 Matrix/8, Create 3x3 Matrix/7, Create 3x3 Matrix/6, Create 3x3 Matrix/4, Create 3x3 Matrix/3, Create 3x3 Matrix/2, Create 3x3 Matrix2/9, Create 3x3 Matrix2/8, Create 3x3 Matrix2/7, Create 3x3 Matrix2/6, Create 3x3 Matrix2/5, Create 3x3 Matrix2/4, Create 3x3 Matrix2/3, Create 3x3 Matrix2/2, Create 3x3 Matrix2/1
  Create 3x3 Matrix1/1 -> Mux/2
  Create 3x3 Matrix/1 -> Mux/1
  Constant9/1 -> Create 3x3 Matrix/5, Create 3x3 Matrix/1, Create 3x3 Matrix/9
  rg_y/1 -> Out3/1
  rg_x/1 -> Out2/1
  Izz/1 -> I_g/9
  Iyy/1 -> I_g/5
  Constant3/1 -> I_g/6
  Constant2/1 -> I_g/4
  Constant5/1 -> I_g/8
  Constant/1 -> I_g/2
  rg_z/1 -> Out4/1
  Ixx/1 -> I_g/1
  Constant4/1 -> I_g/7
  Constant1/1 -> I_g/3

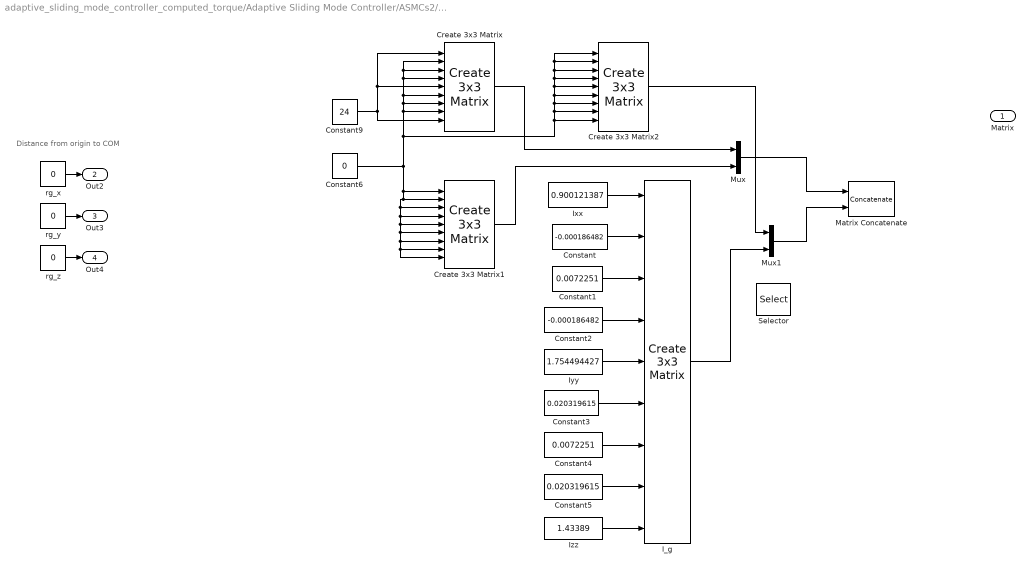
== system adaptive_sliding_mode_controller_computed_torque/Adaptive Sliding Mode Controller/ASMCs2/Subsystem ==
  note: Distance from origin to COM
  Constant : Constant  Value=-0.000186482
  Constant1 : Constant  Value=0.0072251
  Constant2 : Constant  Value=-0.000186482
  Constant3 : Constant  Value=0.020319615
  Constant4 : Constant  Value=0.0072251
  Constant5 : Constant  Value=0.020319615
  Constant6 : Constant  Value=0
  Constant9 : Constant  Value=24
  Create 3x3 Matrix : sharedutil/Create 3x3 Matrix  aMode=aMode
      settings: SourceProductBaseCode=AE,PW,MT,VE,VP
  Create 3x3 Matrix1 : sharedutil/Create 3x3 Matrix  aMode=aMode
      settings: SourceProductBaseCode=AE,PW,MT,VE,VP
  Create 3x3 Matrix2 : sharedutil/Create 3x3 Matrix  aMode=aMode
      settings: SourceProductBaseCode=AE,PW,MT,VE,VP
  I_g : sharedutil/Create 3x3 Matrix  aMode=aMode
      settings: SourceProductBaseCode=AE,PW,MT,VE,VP
  Ixx : Constant  Value=0.900121387
  Iyy : Constant  Value=1.754494427
  Izz : Constant  Value=1.43389
  Matrix Concatenate : Concatenate  Mode=Multidimensional array  ConcatenateDimension=2
  Mux : Mux  Inputs=2
  Mux1 : Mux  Inputs=2
  Selector : Selector  InputPortWidth=3  IndexOptions=Index vector (dialog)  Indices=[1 3]  OutputSizes=1
  rg_x : Constant  Value=0
  rg_y : Constant  Value=0
  rg_z : Constant  Value=0
  Matrix : Outport
  Out2 : Outport  Port=2
  Out3 : Outport  Port=3
  Out4 : Outport  Port=4
  wires:
  Constant1/1 -> I_g/3
  Constant4/1 -> I_g/7
  Ixx/1 -> I_g/1
  rg_z/1 -> Out4/1
  Constant/1 -> I_g/2
  Constant5/1 -> I_g/8
  Constant2/1 -> I_g/4
  Constant3/1 -> I_g/6
  Iyy/1 -> I_g/5
  Izz/1 -> I_g/9
  rg_x/1 -> Out2/1
  rg_y/1 -> Out3/1
  Constant9/1 -> Create 3x3 Matrix/9, Create 3x3 Matrix/1, Create 3x3 Matrix/5
  Create 3x3 Matrix/1 -> Mux/1
  Create 3x3 Matrix1/1 -> Mux/2
  Constant6/1 -> Create 3x3 Matrix2/1, Create 3x3 Matrix2/2, Create 3x3 Matrix2/3, Create 3x3 Matrix2/4, Create 3x3 Matrix2/5, Create 3x3 Matrix2/6, Create 3x3 Matrix2/7, Create 3x3 Matrix2/8, Create 3x3 Matrix2/9, Create 3x3 Matrix/2, Create 3x3 Matrix/3, Create 3x3 Matrix/4, Create 3x3 Matrix/6, Create 3x3 Matrix/7, Create 3x3 Matrix/8, Create 3x3 Matrix1/2, Create 3x3 Matrix1/3, Create 3x3 Matrix1/8, Create 3x3 Matrix1/9, Create 3x3 Matrix1/7, Create 3x3 Matrix1/6, Create 3x3 Matrix1/5, Create 3x3 Matrix1/4, Create 3x3 Matrix1/1
  Create 3x3 Matrix2/1 -> Mux1/1
  I_g/1 -> Mux1/2
  Mux/1 -> Matrix Concatenate/1
  Mux1/1 -> Matrix Concatenate/2

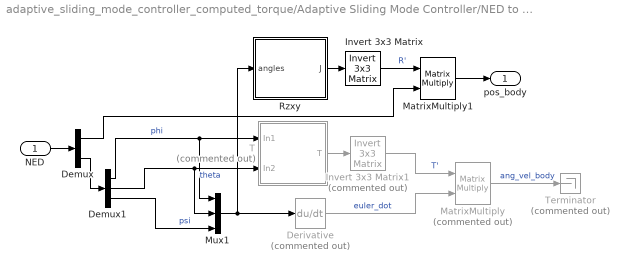
== system adaptive_sliding_mode_controller_computed_torque/Adaptive Sliding Mode Controller/NED to body/Subsystem1 ==
  NED : Inport
  Demux : Demux  Outputs=2
  Demux1 : Demux  Outputs=3
  Derivative : Derivative  Commented=on
  Invert 3x3 Matrix : aerolibutil/Invert  3x3 Matrix
  Invert 3x3 Matrix1 : aerolibutil/Invert  3x3 Matrix  Commented=on
  MatrixMultiply : Product  Commented=on  Multiplication=Matrix(*)
  MatrixMultiply1 : Product  Multiplication=Matrix(*)
  Mux1 : Mux  Inputs=3
  Rzxy : Subsystem
  T : Subsystem  Commented=on
  Terminator : Terminator  Commented=on
  pos_body : Outport
  wires:
  Demux1/2 -> Mux1/2, T/2(In2)  "theta"
  Demux1/1 -> Mux1/1, T/1(In1)  "phi"
  Rzxy/1(J) -> Invert 3x3 Matrix/1
  Mux1/1 -> Derivative/1, Rzxy/1(angles)
  Derivative/1 -> MatrixMultiply/2  "euler_dot"
  Invert 3x3 Matrix1/1 -> MatrixMultiply/1  "T'"
  Demux1/3 -> Mux1/3  "psi"
  MatrixMultiply/1 -> Terminator/1  "ang_vel_body"
  T/1(T) -> Invert 3x3 Matrix1/1
  Invert 3x3 Matrix/1 -> MatrixMultiply1/1  "R'"
  MatrixMultiply1/1 -> pos_body/1
  NED/1 -> Demux/1
  Demux/2 -> Demux1/1
  Demux/1 -> MatrixMultiply1/2

== system adaptive_sliding_mode_controller_computed_torque/Adaptive Sliding Mode Controller/NED to body/Subsystem2 ==
  NED : Inport
  Demux : Demux  Outputs=2
  Demux1 : Demux  Outputs=3
  Derivative : Derivative  Commented=on
  Invert 3x3 Matrix : aerolibutil/Invert  3x3 Matrix
  Invert 3x3 Matrix1 : aerolibutil/Invert  3x3 Matrix  Commented=on
  MatrixMultiply : Product  Commented=on  Multiplication=Matrix(*)
  MatrixMultiply1 : Product  Multiplication=Matrix(*)
  Mux1 : Mux  Inputs=3
  Rzxy : Subsystem
  T : Subsystem  Commented=on
  Terminator : Terminator  Commented=on
  pos_body : Outport
  wires:
  Demux1/2 -> Mux1/2, T/2(In2)  "theta"
  Demux1/1 -> Mux1/1, T/1(In1)  "phi"
  Rzxy/1(J) -> Invert 3x3 Matrix/1
  Mux1/1 -> Derivative/1, Rzxy/1(angles)
  Derivative/1 -> MatrixMultiply/2  "euler_dot"
  Invert 3x3 Matrix1/1 -> MatrixMultiply/1  "T'"
  Demux1/3 -> Mux1/3  "psi"
  MatrixMultiply/1 -> Terminator/1  "ang_vel_body"
  T/1(T) -> Invert 3x3 Matrix1/1
  Invert 3x3 Matrix/1 -> MatrixMultiply1/1  "R'"
  MatrixMultiply1/1 -> pos_body/1
  NED/1 -> Demux/1
  Demux/2 -> Demux1/1
  Demux/1 -> MatrixMultiply1/2

== system adaptive_sliding_mode_controller_computed_torque/Adaptive Sliding Mode Controller/NED to body/Subsystem1/Rzxy ==
  angles : Inport
  3-2-1 convention : Product  Inputs=3  Multiplication=Matrix(*)
  Demux : Demux  Outputs=3
  MATLAB Function1 : MATLAB Function  TreatAsAtomicUnit=on
  MATLAB Function2 : MATLAB Function  TreatAsAtomicUnit=on
  MATLAB Function3 : MATLAB Function  TreatAsAtomicUnit=on
  J : Outport
  wires:
  Demux/1 -> MATLAB Function1/1(phi)
  MATLAB Function3/1(Rz) -> 3-2-1 convention/1
  MATLAB Function2/1(Ry) -> 3-2-1 convention/2
  Demux/3 -> MATLAB Function3/1(psi)
  MATLAB Function1/1(Rx) -> 3-2-1 convention/3
  3-2-1 convention/1 -> J/1
  angles/1 -> Demux/1
  Demux/2 -> MATLAB Function2/1(theta)

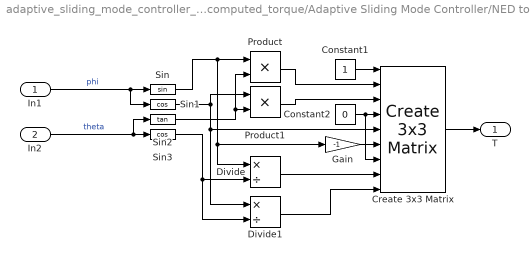
== system adaptive_sliding_mode_controller_computed_torque/Adaptive Sliding Mode Controller/NED to body/Subsystem1/T ==
  In1 : Inport
  In2 : Inport  Port=2
  Constant1 : Constant
  Constant2 : Constant  Value=0
  Create 3x3 Matrix : sharedutil/Create 3x3 Matrix  aMode=aMode
      settings: SourceProductBaseCode=AE,PW,MT,VE,VP
  Divide : Product  Inputs=*/
  Divide1 : Product  Inputs=*/
  Gain : Gain  Gain=-1
  Product : Product
  Product1 : Product
  Sin : Trigonometry
  Sin1 : Trigonometry  Operator=cos
  Sin2 : Trigonometry  Operator=tan
  Sin3 : Trigonometry  Operator=cos
  T : Outport
  wires:
  Constant2/1 -> Create 3x3 Matrix/7, Create 3x3 Matrix/4
  Create 3x3 Matrix/1 -> T/1
  Gain/1 -> Create 3x3 Matrix/6
  Divide1/1 -> Create 3x3 Matrix/9
  Product/1 -> Create 3x3 Matrix/2
  Sin1/1 -> Divide1/1, Create 3x3 Matrix/5, Product1/1
  In1/1 -> Sin1/1, Sin/1  "phi"
  Sin2/1 -> Product/2, Product1/2
  Divide/1 -> Create 3x3 Matrix/8
  Product1/1 -> Create 3x3 Matrix/3
  Sin3/1 -> Divide1/2, Divide/2
  In2/1 -> Sin2/1, Sin3/1  "theta"
  Sin/1 -> Gain/1, Divide/1, Product/1
  Constant1/1 -> Create 3x3 Matrix/1

== system adaptive_sliding_mode_controller_computed_torque/Adaptive Sliding Mode Controller/NED to body/Subsystem2/Rzxy ==
  angles : Inport
  3-2-1 convention : Product  Inputs=3  Multiplication=Matrix(*)
  Demux : Demux  Outputs=3
  MATLAB Function1 : MATLAB Function  TreatAsAtomicUnit=on
  MATLAB Function2 : MATLAB Function  TreatAsAtomicUnit=on
  MATLAB Function3 : MATLAB Function  TreatAsAtomicUnit=on
  J : Outport
  wires:
  Demux/1 -> MATLAB Function1/1(phi)
  MATLAB Function3/1(Rz) -> 3-2-1 convention/1
  MATLAB Function2/1(Ry) -> 3-2-1 convention/2
  Demux/3 -> MATLAB Function3/1(psi)
  MATLAB Function1/1(Rx) -> 3-2-1 convention/3
  3-2-1 convention/1 -> J/1
  angles/1 -> Demux/1
  Demux/2 -> MATLAB Function2/1(theta)

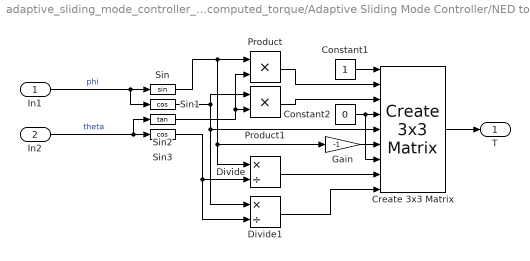
== system adaptive_sliding_mode_controller_computed_torque/Adaptive Sliding Mode Controller/NED to body/Subsystem2/T ==
  In1 : Inport
  In2 : Inport  Port=2
  Constant1 : Constant
  Constant2 : Constant  Value=0
  Create 3x3 Matrix : sharedutil/Create 3x3 Matrix  aMode=aMode
      settings: SourceProductBaseCode=AE,PW,MT,VE,VP
  Divide : Product  Inputs=*/
  Divide1 : Product  Inputs=*/
  Gain : Gain  Gain=-1
  Product : Product
  Product1 : Product
  Sin : Trigonometry
  Sin1 : Trigonometry  Operator=cos
  Sin2 : Trigonometry  Operator=tan
  Sin3 : Trigonometry  Operator=cos
  T : Outport
  wires:
  Constant2/1 -> Create 3x3 Matrix/7, Create 3x3 Matrix/4
  Create 3x3 Matrix/1 -> T/1
  Gain/1 -> Create 3x3 Matrix/6
  Divide1/1 -> Create 3x3 Matrix/9
  Product/1 -> Create 3x3 Matrix/2
  Sin1/1 -> Divide1/1, Create 3x3 Matrix/5, Product1/1
  In1/1 -> Sin1/1, Sin/1  "phi"
  Sin2/1 -> Product/2, Product1/2
  Divide/1 -> Create 3x3 Matrix/8
  Product1/1 -> Create 3x3 Matrix/3
  Sin3/1 -> Divide1/2, Divide/2
  In2/1 -> Sin2/1, Sin3/1  "theta"
  Sin/1 -> Gain/1, Divide/1, Product/1
  Constant1/1 -> Create 3x3 Matrix/1

== matlab function adaptive_sliding_mode_controller_computed_torque/Adaptive Sliding Mode Controller/NED to body/Subsystem1/Rzxy/MATLAB Function2 ==
  data: theta input; Ry output
function Ry = Ry(theta)
Ry = [ cos(theta) 0 sin(theta);
       0          1     0 ;
       -sin(theta) 0 cos(theta); ];

== matlab function adaptive_sliding_mode_controller_computed_torque/Adaptive Sliding Mode Controller/NED to body/Subsystem1/Rzxy/MATLAB Function3 ==
  data: psi input; Rz output
function Rz = Rz(psi)
Rz = [ cos(psi) -sin(psi) 0;
       sin(psi) cos(psi)  0;
       0        0         1];

== matlab function adaptive_sliding_mode_controller_computed_torque/Adaptive Sliding Mode Controller/Thrust allocation/MATLAB Function1 ==
  data: tau input; thrust output; alpha input; rx_v input; ry_v input; unused input; rx_h input; ry_h input; rz_h input
function thrust = thrust_allocation(tau, alpha, rx_v, ry_v, ~, rx_h, ry_h, rz_h)
% Mapping matrix
T = [cos(alpha) cos(alpha) -cos(alpha) -cos(alpha) 0 0;
     -sin(alpha) sin(alpha) -sin(alpha) sin(alpha) 0 0;
     0 0 0 0 -1 -1;
     -sin(alpha)*rz_h sin(alpha)*rz_h -sin(alpha)*rz_h sin(alpha)*rz_h -ry_v ry_v;
     -cos(alpha)*rz_h -cos(alpha)*rz_h cos(alpha)*rz_h cos(alpha)*rz_h -rx_v rx_v;
     -(rx_h*sin(alpha)+ry_h*cos(alpha)) (rx_h*sin(alpha)+ry_h*cos(alpha)) (rx_h*sin(alpha)+ry_h*cos(alpha)) -(rx_h*sin(alpha)+ry_h*cos(alpha)) 0 0
    ];
% Control input with Moore–Penrose pseudo-inverse
t = pinv(T)*tau;
thrust = t;

== matlab function adaptive_sliding_mode_controller_computed_torque/Adaptive Sliding Mode Controller/ASMCs1/MATLAB Function ==
  data: Ma output; in input
function Ma = M(in)
Ma = [0;0;0;0;0;0];
% Skew symmetric matrix
S = @(s) [0    -s(3) s(2);
          s(3) 0     -s(1);
          -s(2) s(1)  0    ];  

% Vehicle parameters
m = 24;

r_g = [0 0 0].';    % Distance from origin to center of mass
I_g = [0.900121387  -0.000186482 0.0072251;
       -0.000186482 1.754494427  0.020319615;
       0.0072251    0.020319615  1.43389     ]; % Rigid-body inertia matrix

% Rigid-Body Inertia Matrix
M_rb = [ m*eye(3)    -m*S(r_g);
         m*S(r_g)         I_g ];

% Added mass matrix
M_a = diag([16.8374 20.2748 35.3180 0.2165 0.6869 0.6157]);

% Mass matrix
Ma = (M_rb + M_a)*in;

== matlab function adaptive_sliding_mode_controller_computed_torque/Adaptive Sliding Mode Controller/ASMCs1/MATLAB Function1 ==
  data: Cv output; vel input
function Cv = C(vel)
v = [0;0;0;0;0;0];
% Skew symmetric matrix
S = @(s) [0    -s(3) s(2);
          s(3) 0     -s(1);
          -s(2) s(1)  0    ];  

% Vehicle parameters
m = 24;

r_g = [0 0 0].';    % Distance from origin to center of mass
I_g = [0.900121387  -0.000186482 0.0072251;
       -0.000186482 1.754494427  0.020319615;
       0.0072251    0.020319615  1.43389     ]; % Rigid-body inertia matrix

% Added mass matrix
M_a = diag([16.8374 20.2748 35.3180 0.2165 0.6869 0.6157]);

%------------ UUV dynamic model parametrization ----------------%
% Rigid-body Coriolis-centripetal Matrix
C_rb = [ zeros(3)             -m*S(vel(1:3))-m*S(vel(4:6))*S(r_g);
        -m*S(vel(1:3))+m*S(r_g)*S(vel(4:6))            -S(I_g*vel(4:6))];

% Coreolis added mass matrix 
C_a = [ 0 0 0   0 -M_a(3,3)*vel(3) M_a(2,2)*vel(2) ;
        0 0 0   M_a(3,3)*vel(3) 0 -M_a(1,1)*vel(1) ;
        0 0 0  -M_a(2,2)*vel(2) M_a(1,1)*vel(1) 0  ;
        0 -M_a(3,3)*vel(3) M_a(2,2)*vel(2)  0 -M_a(6,6)*vel(6) M_a(5,5)*vel(5) ;
        M_a(3,3)*vel(3) 0 -M_a(1,1)*vel(1)  M_a(6,6)*vel(6) 0 -M_a(4,4)*vel(4) ;
       -M_a(2,2)*vel(2) M_a(1,1)*vel(1) 0   -M_a(5,5)*vel(5) M_a(4,4)*vel(4) 0  ];
v = vel;
% Coreolis matrix
C = C_rb + C_a;
Cv = C*v;

== matlab function adaptive_sliding_mode_controller_computed_torque/Adaptive Sliding Mode Controller/ASMCs1/MATLAB Function2 ==
  data: phi input; theta input; g_eta output; unused input
function g_eta = g_eta(phi, theta, ~)
%Fossen (2011): According to (2.2), the sign of the restoring forces and moments fbi 
%and mbi = rbi × fbi , i ∈ {g, b}, must be changed when moving these terms to the 
%left-hand side of (2.2) that is the vector g(η). Pag 60 Handbook of ...

r_g = [0 0 0].';    % Distance from origin to center of mass
r_b = [0 0 -0.10726].';    % Distance from origin to center of buoyancy
m = 24;
W = m*9.81;
B = W*1.005; 
% Restoring forces
g_eta = [ (W-B)*sin(theta);
          -(W-B)*cos(theta)*sin(phi);
          -(W-B)*cos(theta)*cos(phi);
          -(r_g(2)*W-r_b(2)*B)*cos(theta)*cos(phi) + (r_g(3)*W-r_b(3)*B)*cos(theta)*sin(phi);
           (r_g(3)*W-r_b(3)*B)*sin(theta)             + (r_g(1)*W-r_b(1)*B)*cos(theta)*cos(phi)
          -(r_g(1)*W-r_b(1)*B)*cos(theta)*sin(phi) - (r_g(2)*W-r_b(2)*B)*sin(theta)          ];

== matlab function adaptive_sliding_mode_controller_computed_torque/Adaptive Sliding Mode Controller/ASMCs/MATLAB Function ==
  data: Ma output; in input
function Ma = M(in)
Ma = [0;0;0;0;0;0];
% Skew symmetric matrix
S = @(s) [0    -s(3) s(2);
          s(3) 0     -s(1);
          -s(2) s(1)  0    ];  

% Vehicle parameters
m = 24;

r_g = [0 0 0].';    % Distance from origin to center of mass
I_g = [0.900121387  -0.000186482 0.0072251;
       -0.000186482 1.754494427  0.020319615;
       0.0072251    0.020319615  1.43389     ]; % Rigid-body inertia matrix

% Rigid-Body Inertia Matrix
M_rb = [ m*eye(3)    -m*S(r_g);
         m*S(r_g)         I_g ];

% Added mass matrix
M_a = diag([16.8374 20.2748 35.3180 0.2165 0.6869 0.6157]);

% Mass matrix
Ma = (M_rb + M_a)*in;

== matlab function adaptive_sliding_mode_controller_computed_torque/Adaptive Sliding Mode Controller/ASMCs/MATLAB Function1 ==
  data: Cv output; vel input
function Cv = C(vel)
v = [0;0;0;0;0;0];
% Skew symmetric matrix
S = @(s) [0    -s(3) s(2);
          s(3) 0     -s(1);
          -s(2) s(1)  0    ];  

% Vehicle parameters
m = 24;

r_g = [0 0 0].';    % Distance from origin to center of mass
I_g = [0.900121387  -0.000186482 0.0072251;
       -0.000186482 1.754494427  0.020319615;
       0.0072251    0.020319615  1.43389     ]; % Rigid-body inertia matrix

% Added mass matrix
M_a = diag([16.8374 20.2748 35.3180 0.2165 0.6869 0.6157]);

%------------ UUV dynamic model parametrization ----------------%
% Rigid-body Coriolis-centripetal Matrix
C_rb = [ zeros(3)             -m*S(vel(1:3))-m*S(vel(4:6))*S(r_g);
        -m*S(vel(1:3))+m*S(r_g)*S(vel(4:6))            -S(I_g*vel(4:6))];

% Coreolis added mass matrix 
C_a = [ 0 0 0   0 -M_a(3,3)*vel(3) M_a(2,2)*vel(2) ;
        0 0 0   M_a(3,3)*vel(3) 0 -M_a(1,1)*vel(1) ;
        0 0 0  -M_a(2,2)*vel(2) M_a(1,1)*vel(1) 0  ;
        0 -M_a(3,3)*vel(3) M_a(2,2)*vel(2)  0 -M_a(6,6)*vel(6) M_a(5,5)*vel(5) ;
        M_a(3,3)*vel(3) 0 -M_a(1,1)*vel(1)  M_a(6,6)*vel(6) 0 -M_a(4,4)*vel(4) ;
       -M_a(2,2)*vel(2) M_a(1,1)*vel(1) 0   -M_a(5,5)*vel(5) M_a(4,4)*vel(4) 0  ];
v = vel;
% Coreolis matrix
C = C_rb + C_a;
Cv = C*v;

== matlab function adaptive_sliding_mode_controller_computed_torque/Adaptive Sliding Mode Controller/ASMCs/MATLAB Function2 ==
  data: phi input; theta input; g_eta output; unused input
function g_eta = g_eta(phi, theta, ~)
%Fossen (2011): According to (2.2), the sign of the restoring forces and moments fbi 
%and mbi = rbi × fbi , i ∈ {g, b}, must be changed when moving these terms to the 
%left-hand side of (2.2) that is the vector g(η). Pag 60 Handbook of ...

r_g = [0 0 0].';    % Distance from origin to center of mass
r_b = [0 0 -0.10726].';    % Distance from origin to center of buoyancy
m = 24;
W = m*9.81;
B = W*1.005; 
% Restoring forces
g_eta = [ (W-B)*sin(theta);
          -(W-B)*cos(theta)*sin(phi);
          -(W-B)*cos(theta)*cos(phi);
          -(r_g(2)*W-r_b(2)*B)*cos(theta)*cos(phi) + (r_g(3)*W-r_b(3)*B)*cos(theta)*sin(phi);
           (r_g(3)*W-r_b(3)*B)*sin(theta)             + (r_g(1)*W-r_b(1)*B)*cos(theta)*cos(phi)
          -(r_g(1)*W-r_b(1)*B)*cos(theta)*sin(phi) - (r_g(2)*W-r_b(2)*B)*sin(theta)          ];

== matlab function adaptive_sliding_mode_controller_computed_torque/Adaptive Sliding Mode Controller/ASMCs2/MATLAB Function ==
  data: Ma output; in input
function Ma = M(in)
Ma = [0;0;0;0;0;0];
% Skew symmetric matrix
S = @(s) [0    -s(3) s(2);
          s(3) 0     -s(1);
          -s(2) s(1)  0    ];  

% Vehicle parameters
m = 24;

r_g = [0 0 0].';    % Distance from origin to center of mass
I_g = [0.900121387  -0.000186482 0.0072251;
       -0.000186482 1.754494427  0.020319615;
       0.0072251    0.020319615  1.43389     ]; % Rigid-body inertia matrix

% Rigid-Body Inertia Matrix
M_rb = [ m*eye(3)    -m*S(r_g);
         m*S(r_g)         I_g ];

% Added mass matrix
M_a = diag([16.8374 20.2748 35.3180 0.2165 0.6869 0.6157]);

% Mass matrix
Ma = (M_rb + M_a)*in;
